simulink library "csci_gsse_mtv_lib"  (R2014b)
settings: Solver=ode45  StartTime=0.0  StopTime=10.0  RelTol=1e-3
libraries: util_common_lib x2, util_info_lib x1, csc_gnd_sta_lib x1, csc_sim_mtv_simulation_lib x1, csc_valvesim_collection_mtv_lib x1, csu_cfe_cfe_time_lib x1, csu_tlm_telemetry_lib x1, csu_mems_mcu_signal_interface_lib x1, csu_tracker_mcu_signal_interface_lib x1, csu_valvesim_signal_interface_mtv_lib x1
settings Model: Creator=mstewart  LastModifiedBy=mstewart

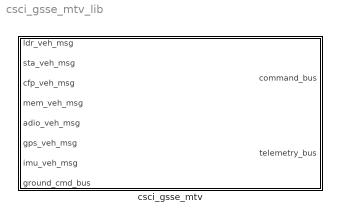
== system csci_gsse_mtv_lib ==
  csci_gsse_mtv : Subsystem

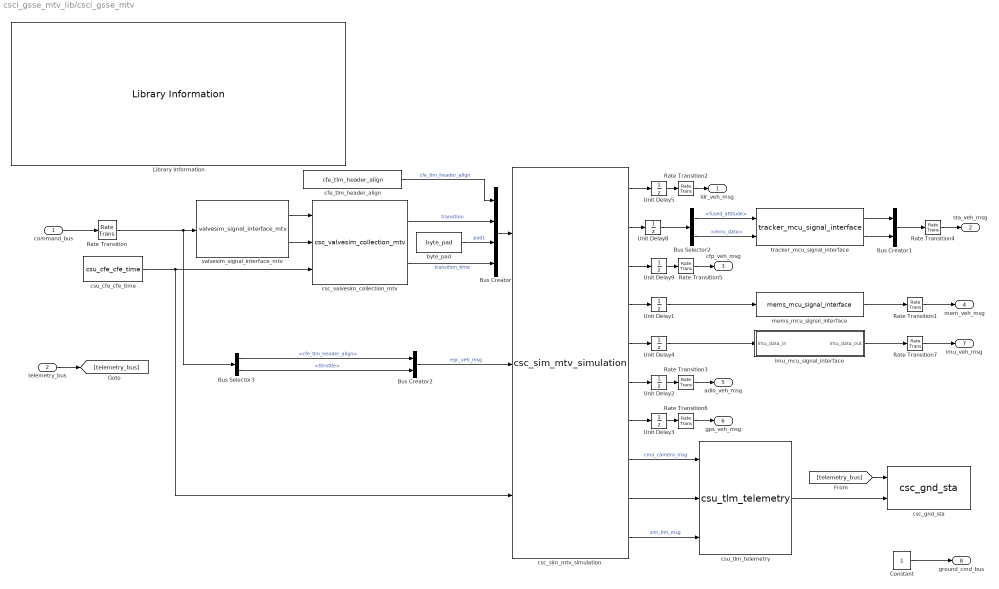
== system csci_gsse_mtv_lib/csci_gsse_mtv ==
  command_bus : Inport
  telemetry_bus : Inport  Port=2
  Bus Creator : BusCreator  OutDataTypeStr=Bus: thr_sim_msg  NonVirtualBus=on
  Bus Creator2 : BusCreator  Inputs=2  OutDataTypeStr=Bus: egc_veh_msg  NonVirtualBus=on
  Bus Selector2 : BusSelector  OutputSignals=fused_attitude,miru_data
  Bus Selector3 : BusSelector  OutputSignals=egc_bus_msg.cfe_tlm_header_align,egc_bus_msg.throttle
  Bus Creator1 : BusCreator  Inputs=2
  Constant : Constant
  Library Information : util_info_lib/Library Information  owner='NONE'
  Rate Transition{,1..7} (8 alike) : RateTransition  Integrity=off
  Unit Delay{1..5,8..9} (7 alike) : UnitDelay  SampleTime=-1
  byte_pad : util_common_lib/byte_pad  n_bytes=6
  cfe_tlm_header_align : util_common_lib/cfe_tlm_header_align
  csc_gnd_sta : csc_gnd_sta_lib/csc_gnd_sta  dir_name=scenario_data_dir
  csc_sim_mtv_simulation : csc_sim_mtv_simulation_lib/csc_sim_mtv_simulation  Tag=GSSE; MDL_TICK=THR_SIM_MSG
  csc_valvesim_collection_mtv : csc_valvesim_collection_mtv_lib/csc_valvesim_collection_mtv  SystemSampleTime=-1
  csu_cfe_cfe_time : csu_cfe_cfe_time_lib/csu_cfe_cfe_time  sch_dt=sim_time_step_size
  csu_tlm_telemetry : csu_tlm_telemetry_lib/csu_tlm_telemetry  num_inputs=3  output_bus_name=sim_telemetry_bus_msg
  imu_mcu_signal_interface : Subsystem
  mems_mcu_signal_interface : csu_mems_mcu_signal_interface_lib/mems_mcu_signal_interface
  tracker_mcu_signal_interface : csu_tracker_mcu_signal_interface_lib/tracker_mcu_signal_interface
  valvesim_signal_interface_mtv : csu_valvesim_signal_interface_mtv_lib/valvesim_signal_interface_mtv
  ldr_veh_msg : Outport
  sta_veh_msg : Outport  Port=2
  cfp_veh_msg : Outport  Port=3
  mem_veh_msg : Outport  Port=4
  adio_veh_msg : Outport  Port=5
  gps_veh_msg : Outport  Port=6
  imu_veh_msg : Outport  Port=7
  ground_cmd_bus : Outport  Port=8
  wires:
  imu_mcu_signal_interface/1(imu_data_out) -> Rate Transition7/1
  Rate Transition7/1 -> imu_veh_msg/1
  Unit Delay4/1 -> imu_mcu_signal_interface/1(imu_data_in)
  csc_sim_mtv_simulation/5 -> Unit Delay4/1
  csc_sim_mtv_simulation/7 -> Unit Delay3/1
  Rate Transition6/1 -> gps_veh_msg/1
  Unit Delay3/1 -> Rate Transition6/1
  Rate Transition3/1 -> adio_veh_msg/1
  csc_sim_mtv_simulation/6 -> Unit Delay2/1
  Unit Delay2/1 -> Rate Transition3/1
  Bus Selector3/2 -> Bus Creator2/2  "<throttle>"
  Bus Selector3/1 -> Bus Creator2/1  "<cfe_tlm_header_align>"
  mems_mcu_signal_interface/1 -> Rate Transition1/1
  Rate Transition1/1 -> mem_veh_msg/1
  Unit Delay1/1 -> mems_mcu_signal_interface/1
  csc_sim_mtv_simulation/4 -> Unit Delay1/1
  Unit Delay8/1 -> Bus Selector2/1
  Bus Selector2/1 -> tracker_mcu_signal_interface/1  "<fused_attitude>"
  Bus Selector2/2 -> tracker_mcu_signal_interface/2  "<miru_data>"
  tracker_mcu_signal_interface/1 -> Bus Creator1/1
  tracker_mcu_signal_interface/2 -> Bus Creator1/2
  Bus Creator1/1 -> Rate Transition4/1
  valvesim_signal_interface_mtv/2 -> csc_valvesim_collection_mtv/2
  cfe_tlm_header_align/1 -> Bus Creator/1  "cfe_tlm_header_align"
  Bus Creator2/1 -> csc_sim_mtv_simulation/2  "egc_veh_msg"
  Rate Transition/1 -> valvesim_signal_interface_mtv/1, Bus Selector3/1
  byte_pad/1 -> Bus Creator/3  "pad1"
  csu_cfe_cfe_time/1 -> csc_valvesim_collection_mtv/3, csc_sim_mtv_simulation/3
  Bus Creator/1 -> csc_sim_mtv_simulation/1
  csc_valvesim_collection_mtv/2 -> Bus Creator/4  "transition_time"
  csc_valvesim_collection_mtv/1 -> Bus Creator/2  "transition"
  valvesim_signal_interface_mtv/1 -> csc_valvesim_collection_mtv/1
  [telemetry_bus] -> csc_gnd_sta/1
  csu_tlm_telemetry/1 -> csc_gnd_sta/2
  csc_sim_mtv_simulation/10 -> csu_tlm_telemetry/3  "sim_tlm_msg"
  csc_sim_mtv_simulation/8 -> csu_tlm_telemetry/1  "cma_camera_msg"
  csc_sim_mtv_simulation/2 -> Unit Delay8/1
  Rate Transition5/1 -> cfp_veh_msg/1
  Rate Transition4/1 -> sta_veh_msg/1
  Rate Transition2/1 -> ldr_veh_msg/1
  command_bus/1 -> Rate Transition/1
  Constant/1 -> ground_cmd_bus/1
  csc_sim_mtv_simulation/3 -> Unit Delay9/1
  csc_sim_mtv_simulation/1 -> Unit Delay5/1
  Unit Delay5/1 -> Rate Transition2/1
  Unit Delay9/1 -> Rate Transition5/1
  csc_sim_mtv_simulation/9 -> csu_tlm_telemetry/2
  telemetry_bus/1 -> [telemetry_bus]

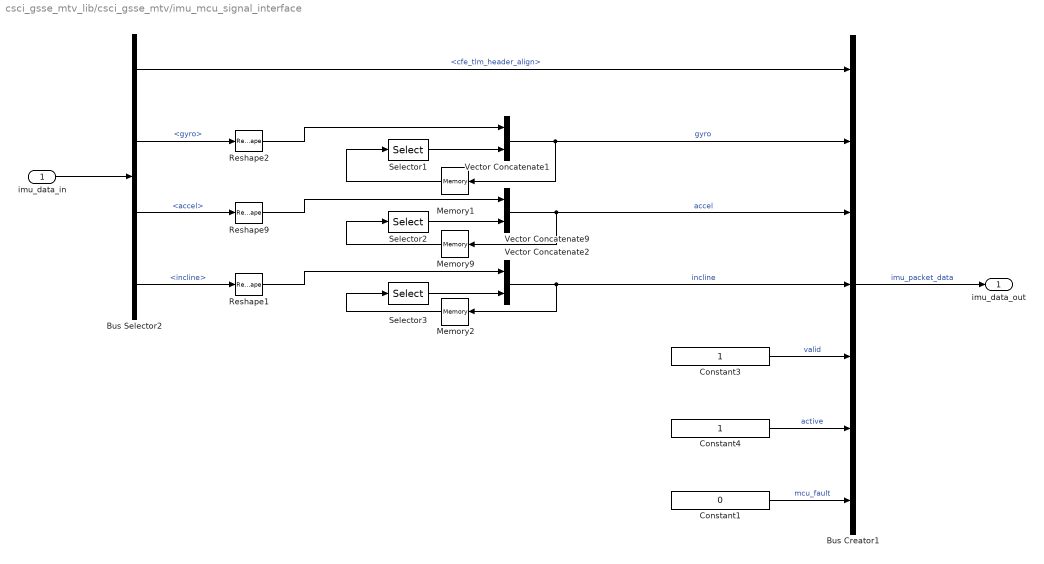
== system csci_gsse_mtv_lib/csci_gsse_mtv/imu_mcu_signal_interface ==
  imu_data_in : Inport
  Bus Selector2 : BusSelector  OutputSignals=cfe_tlm_header_align,gyro,accel,incline
  Bus Creator1 : BusCreator  Inputs=7
  Constant1 : Constant  Value=0  OutDataTypeStr=uint8
  Constant3 : Constant  OutDataTypeStr=uint16
  Constant4 : Constant  OutDataTypeStr=uint8
  Memory1 : Memory  X0=zeros(10,3)  InheritSampleTime=on
  Memory2 : Memory  X0=zeros(10,3)  InheritSampleTime=on
  Memory9 : Memory  X0=zeros(10,3)  InheritSampleTime=on
  Reshape1 : Reshape  OutputDimensionality=Row vector (2-D)
  Reshape2 : Reshape  OutputDimensionality=Row vector (2-D)
  Reshape9 : Reshape  OutputDimensionality=Row vector (2-D)
  Selector1 : Selector  NumberOfDimensions=2  InputPortWidth=10  IndexOptions=Index vector (dialog),Select all  Indices=[1:9],1  OutputSizes=1,1
  Selector2 : Selector  NumberOfDimensions=2  InputPortWidth=10  IndexOptions=Index vector (dialog),Select all  Indices=[1:9],1  OutputSizes=1,1
  Selector3 : Selector  NumberOfDimensions=2  InputPortWidth=10  IndexOptions=Index vector (dialog),Select all  Indices=[1:9],1  OutputSizes=1,1
  Vector Concatenate1 : Concatenate  Mode=Multidimensional array
  Vector Concatenate2 : Concatenate  Mode=Multidimensional array
  Vector Concatenate9 : Concatenate  Mode=Multidimensional array
  imu_data_out : Outport
  wires:
  Bus Selector2/3 -> Reshape9/1  "<accel>"
  Bus Selector2/2 -> Reshape2/1  "<gyro>"
  Constant1/1 -> Bus Creator1/7  "mcu_fault"
  Constant4/1 -> Bus Creator1/6  "active"
  Constant3/1 -> Bus Creator1/5  "valid"
  Reshape9/1 -> Vector Concatenate9/1
  Vector Concatenate9/1 -> Memory9/1, Bus Creator1/3  "accel"
  Selector2/1 -> Vector Concatenate9/2
  Memory9/1 -> Selector2/1
  Reshape2/1 -> Vector Concatenate1/1
  Vector Concatenate1/1 -> Bus Creator1/2, Memory1/1  "gyro"
  Selector1/1 -> Vector Concatenate1/2
  Memory1/1 -> Selector1/1
  imu_data_in/1 -> Bus Selector2/1
  Bus Creator1/1 -> imu_data_out/1  "imu_packet_data"
  Bus Selector2/1 -> Bus Creator1/1  "<cfe_tlm_header_align>"
  Reshape1/1 -> Vector Concatenate2/1
  Vector Concatenate2/1 -> Memory2/1, Bus Creator1/4  "incline"
  Selector3/1 -> Vector Concatenate2/2
  Memory2/1 -> Selector3/1
  Bus Selector2/4 -> Reshape1/1  "<incline>"
